simulink model "Huang_Isoherranen_Mechanistic_Kidney_Model"  (R2017b)
settings: Solver=VariableStepAuto  StartTime=0.0  StopTime=Tfinish  RelTol=1e-3  EnableMultiTasking=on
values from neighbouring files (symbols this model uses):
  alpha_1 = 1    [Huang_Isoherranen_Mechanistic_Kidney_Model_Example_Code.m]
  alpha_10 = 1    [Huang_Isoherranen_Mechanistic_Kidney_Model_Example_Code.m]
  alpha_11 = 1    [Huang_Isoherranen_Mechanistic_Kidney_Model_Example_Code.m]
  alpha_2 = 1    [Huang_Isoherranen_Mechanistic_Kidney_Model_Example_Code.m]
  alpha_3 = 1    [Huang_Isoherranen_Mechanistic_Kidney_Model_Example_Code.m]
  alpha_4 = 1    [Huang_Isoherranen_Mechanistic_Kidney_Model_Example_Code.m]
  alpha_5 = 1    [Huang_Isoherranen_Mechanistic_Kidney_Model_Example_Code.m]
  alpha_6 = 1    [Huang_Isoherranen_Mechanistic_Kidney_Model_Example_Code.m]
  alpha_7 = 1    [Huang_Isoherranen_Mechanistic_Kidney_Model_Example_Code.m]
  alpha_8 = 1    [Huang_Isoherranen_Mechanistic_Kidney_Model_Example_Code.m]
  alpha_9 = 1    [Huang_Isoherranen_Mechanistic_Kidney_Model_Example_Code.m]
  beta = 1    [Huang_Isoherranen_Mechanistic_Kidney_Model_Example_Code.m]
  BP0 = 1    [Huang_Isoherranen_Mechanistic_Kidney_Model_Example_Code.m]
  CL_api_reabs = 0    [Huang_Isoherranen_Mechanistic_Kidney_Model_Example_Code.m]
  CL_BC = 0    [Huang_Isoherranen_Mechanistic_Kidney_Model_Example_Code.m]
  CL_bsl_reabs = 0    [Huang_Isoherranen_Mechanistic_Kidney_Model_Example_Code.m]
  CL_CT = 0    [Huang_Isoherranen_Mechanistic_Kidney_Model_Example_Code.m]
  CL_kidney_intrinsic = 0    [Huang_Isoherranen_Mechanistic_Kidney_Model_Example_Code.m]
  CL_PD_CD = S_CD * Papp    (= 0.01608)    [Huang_Isoherranen_Mechanistic_Kidney_Model_Example_Code.m]
  CL_PD_DS = S_DT * Papp    (= 0.3744)    [Huang_Isoherranen_Mechanistic_Kidney_Model_Example_Code.m]
  CL_PD_LH = S_HT * Papp    (= 0.1464)    [Huang_Isoherranen_Mechanistic_Kidney_Model_Example_Code.m]
  CL_PD_PX_apical = S_PT * Papp    (= 14.6568)    [Huang_Isoherranen_Mechanistic_Kidney_Model_Example_Code.m]
  CL_PD_PX_basolateral = S_PT/30 * Papp    (= 0.48856)    [Huang_Isoherranen_Mechanistic_Kidney_Model_Example_Code.m]
  CLh = 0    [Huang_Isoherranen_Mechanistic_Kidney_Model_Example_Code.m]
  fu0 = 1    [Huang_Isoherranen_Mechanistic_Kidney_Model_Example_Code.m]
  fu_k = fu0    (= 1)    [Huang_Isoherranen_Mechanistic_Kidney_Model_Example_Code.m]
  gamma = 1    [Huang_Isoherranen_Mechanistic_Kidney_Model_Example_Code.m]
  Infusion_length = 240    [Huang_Isoherranen_Mechanistic_Kidney_Model_Example_Code.m]
  IR = 1    [Huang_Isoherranen_Mechanistic_Kidney_Model_Example_Code.m]
  ivbolusDose1 = 0    [Huang_Isoherranen_Mechanistic_Kidney_Model_Example_Code.m]
  ivT1 = 0    [Huang_Isoherranen_Mechanistic_Kidney_Model_Example_Code.m]
  Q_connectingtubule = 11    [Huang_Isoherranen_Mechanistic_Kidney_Model_Example_Code.m]
  Q_corticalCD = 7    [Huang_Isoherranen_Mechanistic_Kidney_Model_Example_Code.m]
  Q_GFR = 7.2    [Huang_Isoherranen_Mechanistic_Kidney_Model_Example_Code.m]
  Q_initialCD = 9    [Huang_Isoherranen_Mechanistic_Kidney_Model_Example_Code.m]
  Q_kidney0 = 60    [Huang_Isoherranen_Mechanistic_Kidney_Model_Example_Code.m]
  Q_medullaryCD = 5    [Huang_Isoherranen_Mechanistic_Kidney_Model_Example_Code.m]
  Q_papillary = 3    [Huang_Isoherranen_Mechanistic_Kidney_Model_Example_Code.m]
  Q_urine = 1    [Huang_Isoherranen_Mechanistic_Kidney_Model_Example_Code.m]
  Qc0 = 330    [Huang_Isoherranen_Mechanistic_Kidney_Model_Example_Code.m]
  Tstart_infusion = 0    [Huang_Isoherranen_Mechanistic_Kidney_Model_Example_Code.m]
  V_CDB = 0.237    [Huang_Isoherranen_Mechanistic_Kidney_Model_Example_Code.m]
  V_CDC = 0.237    [Huang_Isoherranen_Mechanistic_Kidney_Model_Example_Code.m]
  V_CDT = 0.237    [Huang_Isoherranen_Mechanistic_Kidney_Model_Example_Code.m]
  V_DB = 0.0194    [Huang_Isoherranen_Mechanistic_Kidney_Model_Example_Code.m]
  V_DC = 0.0194    [Huang_Isoherranen_Mechanistic_Kidney_Model_Example_Code.m]
  V_DT = 0.0194    [Huang_Isoherranen_Mechanistic_Kidney_Model_Example_Code.m]
  V_HB = 0.0027    [Huang_Isoherranen_Mechanistic_Kidney_Model_Example_Code.m]
  V_HC = 0.0027    [Huang_Isoherranen_Mechanistic_Kidney_Model_Example_Code.m]
  V_HT = 0.0027    [Huang_Isoherranen_Mechanistic_Kidney_Model_Example_Code.m]
  V_PB = 0.0305    [Huang_Isoherranen_Mechanistic_Kidney_Model_Example_Code.m]
  V_PC = 0.0305    [Huang_Isoherranen_Mechanistic_Kidney_Model_Example_Code.m]
  V_PT = 0.0305    [Huang_Isoherranen_Mechanistic_Kidney_Model_Example_Code.m]
  V_ven0 = 42    [Huang_Isoherranen_Mechanistic_Kidney_Model_Example_Code.m]
libraries: simulink x3, dspmathops x1
(part 1 of 2)
settings Model: Creator=Weize Huang  LastModifiedBy=isolab
settings SolverCC: MaxConsecutiveZCs=2000
settings OptimizationCC: LifeSpan=inf
settings DebuggingCC: SFUnexpectedBacktrackingDiag=warning  SFNoUnconditionalDefaultTransitionDiag=warning  SFExecutionAtInitializationDiag=none
settings CodeAppCC: StateflowObjectComments=on
settings GRTTargetCC: TargetLangStandard=C89/C90 (ANSI)  GeneratePreprocessorConditionals=Disable all
settings ConfigComp: CovMetricSettings=dw  CovHtmlReporting=on  CovSaveCumulativeToWorkspaceVar=on  CovSaveSingleToWorkspaceVar=on  CovExternalEMLEnable=off

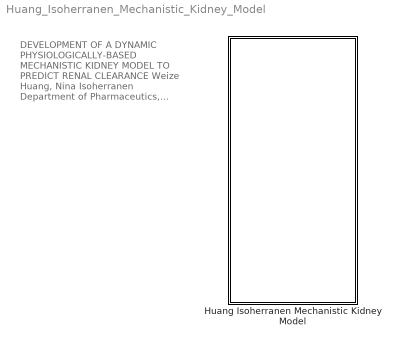
== system Huang_Isoherranen_Mechanistic_Kidney_Model ==
  note: DEVELOPMENT OF A DYNAMIC PHYSIOLOGICALLY-BASED MECHANISTIC KIDNEY MODEL TO PREDICT RENAL CLEARANCE
      | Weize Huang, Nina Isoherranen
      | Department of Pharmaceutics, School of Pharmacy, University of Washington, Seattle, WA, 98195
      | May 2nd 2018
  Huang Isoherranen Mechanistic Kidney Model : Subsystem

== system Huang_Isoherranen_Mechanistic_Kidney_Model/Huang Isoherranen Mechanistic Kidney Model ==
  note: DEVELOPMENT OF A DYNAMIC PHYSIOLOGICALLY-BASED MECHANISTIC KIDNEY MODEL TO PREDICT RENAL CLEARANCE
      | Weize Huang, Nina Isoherranen
      | Department of Pharmaceutics, School of Pharmacy, University of Washington, Seattle, WA, 98195
      | May 2nd 2018
  Kidney : Subsystem
  venous blood : Subsystem
  wires:
  Kidney/1(Out1) -> venous blood/2(In2)
  venous blood/1(Out1) -> Kidney/1(In1), venous blood/1(In1)

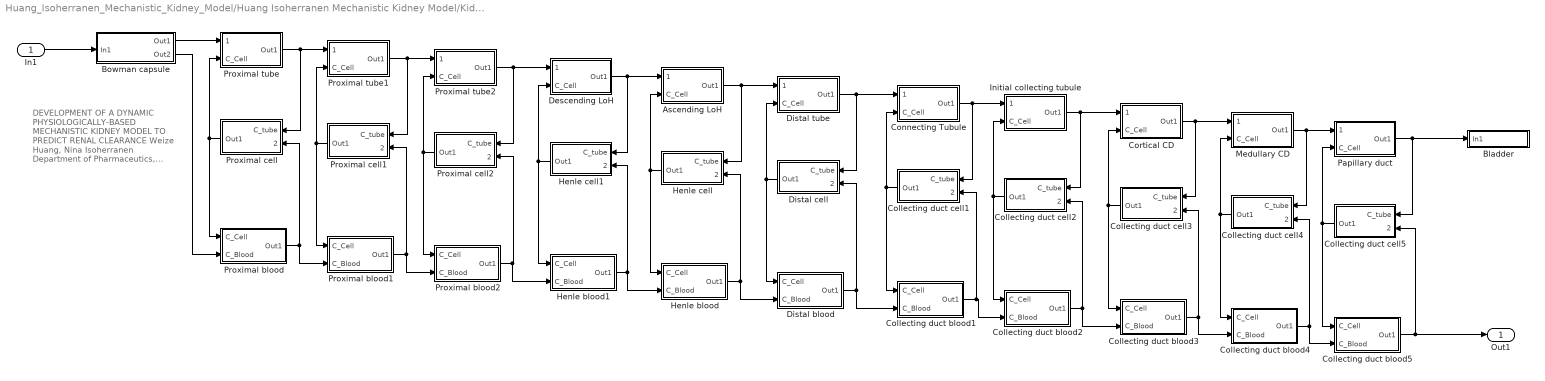
== system Huang_Isoherranen_Mechanistic_Kidney_Model/Huang Isoherranen Mechanistic Kidney Model/Kidney ==
  note: DEVELOPMENT OF A DYNAMIC PHYSIOLOGICALLY-BASED MECHANISTIC KIDNEY MODEL TO PREDICT RENAL CLEARANCE
      | Weize Huang, Nina Isoherranen
      | Department of Pharmaceutics, School of Pharmacy, University of Washington, Seattle, WA, 98195
      | May 2nd 2018
  In1 : Inport
  Ascending LoH : Subsystem
  Bladder : Subsystem
  Bowman capsule : Subsystem
  Collecting duct blood1 : Subsystem
  Collecting duct blood2 : Subsystem
  Collecting duct blood3 : Subsystem
  Collecting duct blood4 : Subsystem
  Collecting duct blood5 : Subsystem
  Collecting duct cell1 : Subsystem
  Collecting duct cell2 : Subsystem
  Collecting duct cell3 : Subsystem
  Collecting duct cell4 : Subsystem
  Collecting duct cell5 : Subsystem
  Connecting Tubule : Subsystem
  Cortical CD : Subsystem
  Descending LoH : Subsystem
  Distal blood : Subsystem
  Distal cell : Subsystem
  Distal tube : Subsystem
  Henle blood : Subsystem
  Henle blood1 : Subsystem
  Henle cell : Subsystem
  Henle cell1 : Subsystem
  Initial collecting tubule : Subsystem
  Medullary CD : Subsystem
  Papillary duct : Subsystem
  Proximal blood : Subsystem
  Proximal blood1 : Subsystem
  Proximal blood2 : Subsystem
  Proximal cell : Subsystem
  Proximal cell1 : Subsystem
  Proximal cell2 : Subsystem
  Proximal tube : Subsystem
  Proximal tube1 : Subsystem
  Proximal tube2 : Subsystem
  Out1 : Outport
  wires:
  In1/1 -> Bowman capsule/1(In1)
  Bowman capsule/1(Out1) -> Proximal tube/1(C_Tube)
  Proximal tube/1(Out1) -> Proximal tube1/1(C_Tube), Proximal cell/1(C_tube)
  Proximal cell/1(Out1) -> Proximal tube/2(C_Cell), Proximal blood/1(C_Cell)
  Proximal blood/1(Out1) -> Proximal blood1/2(C_Blood), Proximal cell/2(C_blood)
  Proximal tube1/1(Out1) -> Proximal cell1/1(C_tube), Proximal tube2/1(C_Tube)
  Proximal blood1/1(Out1) -> Proximal blood2/2(C_Blood), Proximal cell1/2(C_blood)
  Proximal tube2/1(Out1) -> Proximal cell2/1(C_tube), Descending LoH/1(C_Tube)
  Proximal blood2/1(Out1) -> Proximal cell2/2(C_blood), Henle blood1/2(C_Blood)
  Proximal cell1/1(Out1) -> Proximal blood1/1(C_Cell), Proximal tube1/2(C_Cell)
  Proximal cell2/1(Out1) -> Proximal blood2/1(C_Cell), Proximal tube2/2(C_Cell)
  Ascending LoH/1(Out1) -> Distal tube/1(C_Tube), Henle cell/1(C_tube)
  Henle cell/1(Out1) -> Henle blood/1(C_Cell), Ascending LoH/2(C_Cell)
  Henle blood/1(Out1) -> Distal blood/2(C_Blood), Henle cell/2(C_blood)
  Distal tube/1(Out1) -> Distal cell/1(C_tube), Connecting Tubule/1(C_Tube)
  Distal cell/1(Out1) -> Distal blood/1(C_Cell), Distal tube/2(C_Cell)
  Distal blood/1(Out1) -> Distal cell/2(C_blood), Collecting duct blood1/2(C_Blood)
  Collecting duct cell1/1(Out1) -> Collecting duct blood1/1(C_Cell), Connecting Tubule/2(C_Cell)
  Collecting duct cell4/1(Out1) -> Collecting duct blood4/1(C_Cell), Medullary CD/2(C_Cell)
  Collecting duct cell2/1(Out1) -> Collecting duct blood2/1(C_Cell), Initial collecting tubule/2(C_Cell)
  Collecting duct cell3/1(Out1) -> Collecting duct blood3/1(C_Cell), Cortical CD/2(C_Cell)
  Connecting Tubule/1(Out1) -> Collecting duct cell1/1(C_tube), Initial collecting tubule/1(C_Tube)
  Collecting duct blood1/1(Out1) -> Collecting duct cell1/2(C_blood), Collecting duct blood2/2(C_Blood)
  Initial collecting tubule/1(Out1) -> Collecting duct cell2/1(C_tube), Cortical CD/1(C_Tube)
  Collecting duct blood2/1(Out1) -> Collecting duct cell2/2(C_blood), Collecting duct blood3/2(C_Blood)
  Cortical CD/1(Out1) -> Collecting duct cell3/1(C_tube), Medullary CD/1(C_Tube)
  Collecting duct blood3/1(Out1) -> Collecting duct blood4/2(C_Blood), Collecting duct cell3/2(C_blood)
  Henle blood1/1(Out1) -> Henle cell1/2(C_blood), Henle blood/2(C_Blood)
  Papillary duct/1(Out1) -> Collecting duct cell5/1(C_tube), Bladder/1(In1)
  Collecting duct blood5/1(Out1) -> Collecting duct cell5/2(C_blood), Out1/1
  Collecting duct cell5/1(Out1) -> Collecting duct blood5/1(C_Cell), Papillary duct/2(C_Cell)
  Medullary CD/1(Out1) -> Collecting duct cell4/1(C_tube), Papillary duct/1(C_Tube)
  Collecting duct blood4/1(Out1) -> Collecting duct blood5/2(C_Blood), Collecting duct cell4/2(C_blood)
  Henle cell1/1(Out1) -> Henle blood1/1(C_Cell), Descending LoH/2(C_Cell)
  Descending LoH/1(Out1) -> Henle cell1/1(C_tube), Ascending LoH/1(C_Tube)
  Bowman capsule/2(Out2) -> Proximal blood/2(C_Blood)

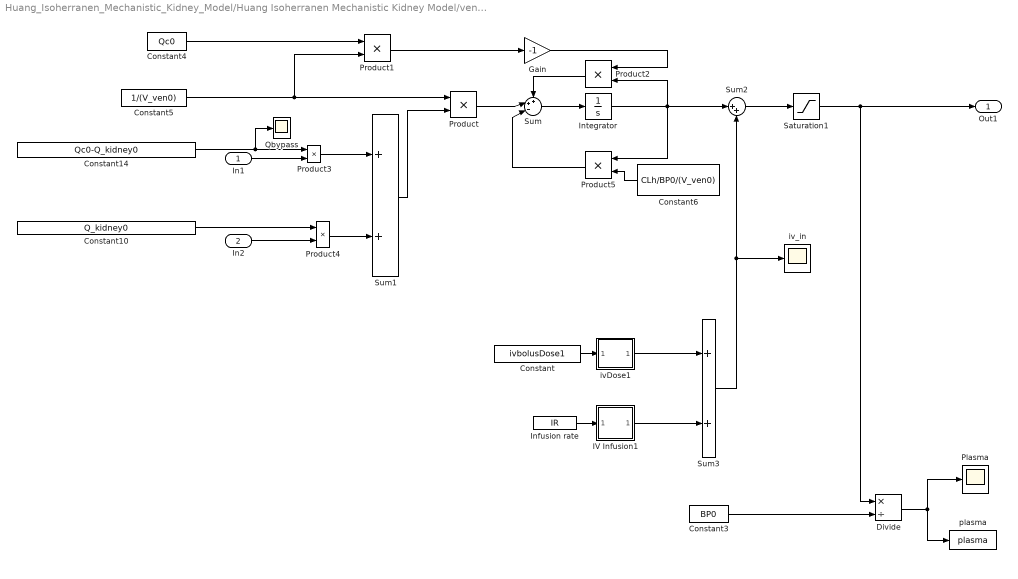
== system Huang_Isoherranen_Mechanistic_Kidney_Model/Huang Isoherranen Mechanistic Kidney Model/venous blood ==
  In1 : Inport
  In2 : Inport  Port=2
  Constant : Constant  Value=ivbolusDose1
  Constant10 : Constant  Value=Q_kidney0
  Constant14 : Constant  Value=Qc0-Q_kidney0
  Constant3 : Constant  Value=BP0
  Constant4 : Constant  Value=Qc0
  Constant5 : Constant  Value=1/(V_ven0)
  Constant6 : Constant  Value=CLh/BP0/(V_ven0)
  Divide : Product  Inputs=*/
  Gain : Gain  Gain=-1
  IV Infusion1 : Subsystem
  Infusion rate : Constant  Value=IR
  Integrator : Integrator
  Plasma : Scope
  Product{,1..5} (6 alike) : Product  RndMeth=Zero
  Qbypass : Scope
  Saturation1 : Saturate  UpperLimit=1000000000  LowerLimit=0
  Sum : Sum  Inputs=++-|
  Sum1 : Sum
  Sum2 : Sum  Inputs=|++
  Sum3 : Sum
  ivDose1 : Subsystem
  iv_in : Scope
  plasma : ToWorkspace  VariableName=plasma  SampleTime=-1
  Out1 : Outport
  wires:
  Product1/1 -> Gain/1
  Product2/1 -> Sum/1
  Product/1 -> Sum/2
  Sum/1 -> Integrator/1
  Gain/1 -> Product2/1
  Sum1/1 -> Product/2
  Sum2/1 -> Saturation1/1
  Product3/1 -> Sum1/1
  Product4/1 -> Sum1/2
  Divide/1 -> plasma/1, Plasma/1
  Constant3/1 -> Divide/2
  Constant10/1 -> Product4/1
  Constant14/1 -> Qbypass/1, Product3/1
  Constant5/1 -> Product/1, Product1/2
  Integrator/1 -> Product5/1, Sum2/1, Product2/2
  Constant4/1 -> Product1/1
  Constant/1 -> ivDose1/1(In1)
  Sum3/1 -> Sum2/2, iv_in/1
  ivDose1/1(Out1) -> Sum3/1
  Saturation1/1 -> Out1/1, Divide/1
  In1/1 -> Product3/2
  In2/1 -> Product4/2
  Constant6/1 -> Product5/2
  Product5/1 -> Sum/3
  Infusion rate/1 -> IV Infusion1/1(In1)
  IV Infusion1/1(Out1) -> Sum3/2

== system Huang_Isoherranen_Mechanistic_Kidney_Model/Huang Isoherranen Mechanistic Kidney Model/Kidney/Ascending LoH ==
  C_Tube : Inport
  C_Cell : Inport  Port=2
  C_HT : ToWorkspace  VariableName=C_HT_2  SampleTime=-1
  Constant1 : Constant  Value=V_HT
  Constant2 : Constant  Value=CL_PD_LH
  Constant3 : Constant  Value=beta
  Constant4 : Constant  Value=Q_GFR/120*24
  Constant5 : Constant  Value=Q_GFR/120*24
  Constant6 : Constant  Value=alpha_5
  Constant7 : Constant  Value=fu_k
  Divide1 : Product  Inputs=/*
  Integrator : Integrator
  Product{,1..3,5} (5 alike) : Product  RndMeth=Zero
  Product6 : Product  Inputs=3  RndMeth=Zero
  Saturation : Saturate  UpperLimit=1000000000  LowerLimit=0
  Subtract : Sum
  Subtract1 : Sum
  Sum : Sum  Inputs=+-|
  scope : Scope
  Out1 : Outport
  wires:
  Integrator/1 -> Product2/2, Product6/3, Saturation/1, scope/1, C_HT/1
  Sum/1 -> Divide1/2
  Saturation/1 -> Out1/1
  C_Tube/1 -> Product/2
  Constant7/1 -> Product1/1
  C_Cell/1 -> Product1/2
  Product1/1 -> Product3/1
  Constant5/1 -> Product/1
  Product3/1 -> Subtract/1
  Product/1 -> Subtract/2
  Constant1/1 -> Divide1/1
  Subtract/1 -> Sum/1
  Divide1/1 -> Integrator/1
  Constant4/1 -> Product2/1
  Constant3/1 -> Product5/1
  Constant2/1 -> Product6/2, Product5/2
  Product5/1 -> Product3/2
  Constant6/1 -> Product6/1
  Product6/1 -> Subtract1/1
  Product2/1 -> Subtract1/2
  Subtract1/1 -> Sum/2

== system Huang_Isoherranen_Mechanistic_Kidney_Model/Huang Isoherranen Mechanistic Kidney Model/Kidney/Bladder ==
  In1 : Inport
  Ae : ToWorkspace  VariableName=Ae  SampleTime=-1
  C_bladder_urine : ToWorkspace  VariableName=C_bladder_urine  SampleTime=-1
  Constant4 : Constant  Value=Q_GFR/120*Q_urine
  Cum_Ae : ToWorkspace  VariableName=Cum_Ae  SampleTime=-1
  Cumulative Sum : dspmathops/Cumulative Sum  dim=Columns  InputProcessing=Columns as channels (frame based)  reset_popup=None  outputDataTypeStr=Inherit: Same as accumulator  outputLastDataTypeStr=Inherit: Same as accumulator  outputMin=[]  outputMax=[]  roundingMode=Floor  overflowMode=off
      settings: SourceProductName=DSP System Toolbox
  Gain : Gain
  Integrator : Integrator
  Product2 : Product  RndMeth=Zero
  scope : Scope
  wires:
  In1/1 -> Gain/1
  Gain/1 -> Product2/1, scope/1, C_bladder_urine/1
  Constant4/1 -> Product2/2
  Product2/1 -> Integrator/1
  Integrator/1 -> Cumulative Sum/1, Ae/1
  Cumulative Sum/1 -> Cum_Ae/1

== system Huang_Isoherranen_Mechanistic_Kidney_Model/Huang Isoherranen Mechanistic Kidney Model/Kidney/Bowman capsule ==
  In1 : Inport
  Bowman : ToWorkspace  VariableName=Bowman  SampleTime=-1
  Constant : Constant  Value=fu0/BP0
  Constant1 : Constant  Value=1-fu0/BP0*Q_GFR/Q_kidney0
  Product1 : Product  RndMeth=Zero
  Product2 : Product  RndMeth=Zero
  Saturation : Saturate  UpperLimit=1000000000  LowerLimit=0
  blood_after_filtration : ToWorkspace  VariableName=C_blood_after_filtration1  SampleTime=-1
  scope : Scope
  scope1 : Scope
  Out1 : Outport
  Out2 : Outport  Port=2
  wires:
  Product1/1 -> scope/1, Bowman/1, Saturation/1
  Saturation/1 -> Out1/1
  In1/1 -> Product2/2, Product1/1
  Constant/1 -> Product1/2
  Product2/1 -> Out2/1, scope1/1, blood_after_filtration/1
  Constant1/1 -> Product2/1

== system Huang_Isoherranen_Mechanistic_Kidney_Model/Huang Isoherranen Mechanistic Kidney Model/Kidney/Collecting duct blood1 ==
  C_Cell : Inport
  C_Blood : Inport  Port=2
  C_CDB_1 : ToWorkspace  VariableName=C_CDB  SampleTime=-1
  Constant : Constant  Value=fu0/BP0
  Constant1 : Constant  Value=V_CDB
  Constant2 : Constant  Value=CL_PD_CD
  Constant3 : Constant  Value=beta
  Constant5 : Constant  Value=Q_kidney0
  Constant6 : Constant  Value=gamma
  Constant7 : Constant  Value=fu_k
  Divide1 : Product  Inputs=/*
  Integrator : Integrator
  Product{,1..3,5} (5 alike) : Product  RndMeth=Zero
  Product6 : Product  Inputs=4  RndMeth=Zero
  Saturation : Saturate  UpperLimit=1000000000  LowerLimit=0
  Subtract : Sum
  Subtract1 : Sum
  Sum : Sum  Inputs=+-|
  scope : Scope
  Out1 : Outport
  wires:
  Integrator/1 -> Product2/2, Product6/4, Saturation/1, scope/1, C_CDB_1/1
  Sum/1 -> Divide1/2
  Saturation/1 -> Out1/1
  Constant7/1 -> Product1/1
  Product1/1 -> Product3/1
  Constant5/1 -> Product2/1, Product/1
  Product3/1 -> Subtract/1
  Product/1 -> Subtract/2
  Constant1/1 -> Divide1/1
  Subtract/1 -> Sum/1
  Divide1/1 -> Integrator/1
  Constant3/1 -> Product5/1
  Constant2/1 -> Product6/3, Product5/2
  Product5/1 -> Product3/2
  Subtract1/1 -> Sum/2
  C_Cell/1 -> Product1/2
  C_Blood/1 -> Product/2
  Constant/1 -> Product6/1
  Product2/1 -> Subtract1/1
  Constant6/1 -> Product6/2
  Product6/1 -> Subtract1/2

== system Huang_Isoherranen_Mechanistic_Kidney_Model/Huang Isoherranen Mechanistic Kidney Model/Kidney/Collecting duct blood2 ==
  C_Cell : Inport
  C_Blood : Inport  Port=2
  C_CDB_2 : ToWorkspace  VariableName=C_CDB_2  SampleTime=-1
  Constant : Constant  Value=fu0/BP0
  Constant1 : Constant  Value=V_CDB
  Constant2 : Constant  Value=CL_PD_CD
  Constant3 : Constant  Value=beta
  Constant5 : Constant  Value=Q_kidney0
  Constant6 : Constant  Value=gamma
  Constant7 : Constant  Value=fu_k
  Divide1 : Product  Inputs=/*
  Integrator : Integrator
  Product{,1..3,5} (5 alike) : Product  RndMeth=Zero
  Product6 : Product  Inputs=4  RndMeth=Zero
  Saturation : Saturate  UpperLimit=1000000000  LowerLimit=0
  Subtract : Sum
  Subtract1 : Sum
  Sum : Sum  Inputs=+-|
  scope : Scope
  Out1 : Outport
  wires:
  Integrator/1 -> Product2/2, Product6/4, Saturation/1, scope/1, C_CDB_2/1
  Sum/1 -> Divide1/2
  Saturation/1 -> Out1/1
  Constant7/1 -> Product1/1
  Product1/1 -> Product3/1
  Constant5/1 -> Product2/1, Product/1
  Product3/1 -> Subtract/1
  Product/1 -> Subtract/2
  Constant1/1 -> Divide1/1
  Subtract/1 -> Sum/1
  Divide1/1 -> Integrator/1
  Constant3/1 -> Product5/1
  Constant2/1 -> Product6/3, Product5/2
  Product5/1 -> Product3/2
  Subtract1/1 -> Sum/2
  C_Cell/1 -> Product1/2
  C_Blood/1 -> Product/2
  Constant/1 -> Product6/1
  Product2/1 -> Subtract1/1
  Constant6/1 -> Product6/2
  Product6/1 -> Subtract1/2

== system Huang_Isoherranen_Mechanistic_Kidney_Model/Huang Isoherranen Mechanistic Kidney Model/Kidney/Collecting duct blood3 ==
  C_Cell : Inport
  C_Blood : Inport  Port=2
  C_CDB_3 : ToWorkspace  VariableName=C_CDB_3  SampleTime=-1
  Constant : Constant  Value=fu0/BP0
  Constant1 : Constant  Value=V_CDB
  Constant2 : Constant  Value=CL_PD_CD
  Constant3 : Constant  Value=beta
  Constant5 : Constant  Value=Q_kidney0
  Constant6 : Constant  Value=gamma
  Constant7 : Constant  Value=fu_k
  Divide1 : Product  Inputs=/*
  Integrator : Integrator
  Product{,1..3,5} (5 alike) : Product  RndMeth=Zero
  Product6 : Product  Inputs=4  RndMeth=Zero
  Saturation : Saturate  UpperLimit=1000000000  LowerLimit=0
  Subtract : Sum
  Subtract1 : Sum
  Sum : Sum  Inputs=+-|
  scope : Scope
  Out1 : Outport
  wires:
  Integrator/1 -> Product2/2, Product6/4, Saturation/1, scope/1, C_CDB_3/1
  Sum/1 -> Divide1/2
  Saturation/1 -> Out1/1
  Constant7/1 -> Product1/1
  Product1/1 -> Product3/1
  Constant5/1 -> Product2/1, Product/1
  Product3/1 -> Subtract/1
  Product/1 -> Subtract/2
  Constant1/1 -> Divide1/1
  Subtract/1 -> Sum/1
  Divide1/1 -> Integrator/1
  Constant3/1 -> Product5/1
  Constant2/1 -> Product6/3, Product5/2
  Product5/1 -> Product3/2
  Subtract1/1 -> Sum/2
  C_Cell/1 -> Product1/2
  C_Blood/1 -> Product/2
  Constant/1 -> Product6/1
  Product2/1 -> Subtract1/1
  Constant6/1 -> Product6/2
  Product6/1 -> Subtract1/2

== system Huang_Isoherranen_Mechanistic_Kidney_Model/Huang Isoherranen Mechanistic Kidney Model/Kidney/Collecting duct blood4 ==
  C_Cell : Inport
  C_Blood : Inport  Port=2
  C_CDB_4 : ToWorkspace  VariableName=C_CDB_4  SampleTime=-1
  Constant : Constant  Value=fu0/BP0
  Constant1 : Constant  Value=V_CDB
  Constant2 : Constant  Value=CL_PD_CD
  Constant3 : Constant  Value=beta
  Constant5 : Constant  Value=Q_kidney0
  Constant6 : Constant  Value=gamma
  Constant7 : Constant  Value=fu_k
  Divide1 : Product  Inputs=/*
  Integrator : Integrator
  Product{,1..3,5} (5 alike) : Product  RndMeth=Zero
  Product6 : Product  Inputs=4  RndMeth=Zero
  Saturation : Saturate  UpperLimit=1000000000  LowerLimit=0
  Subtract : Sum
  Subtract1 : Sum
  Sum : Sum  Inputs=+-|
  scope : Scope
  Out1 : Outport
  wires:
  Integrator/1 -> Product2/2, Product6/4, Saturation/1, scope/1, C_CDB_4/1
  Sum/1 -> Divide1/2
  Saturation/1 -> Out1/1
  Constant7/1 -> Product1/1
  Product1/1 -> Product3/1
  Constant5/1 -> Product2/1, Product/1
  Product3/1 -> Subtract/1
  Product/1 -> Subtract/2
  Constant1/1 -> Divide1/1
  Subtract/1 -> Sum/1
  Divide1/1 -> Integrator/1
  Constant3/1 -> Product5/1
  Constant2/1 -> Product6/3, Product5/2
  Product5/1 -> Product3/2
  Subtract1/1 -> Sum/2
  C_Cell/1 -> Product1/2
  C_Blood/1 -> Product/2
  Constant/1 -> Product6/1
  Product2/1 -> Subtract1/1
  Constant6/1 -> Product6/2
  Product6/1 -> Subtract1/2

== system Huang_Isoherranen_Mechanistic_Kidney_Model/Huang Isoherranen Mechanistic Kidney Model/Kidney/Collecting duct blood5 ==
  C_Cell : Inport
  C_Blood : Inport  Port=2
  C_CDB_4 : ToWorkspace  VariableName=C_CDB_5  SampleTime=-1
  Constant : Constant  Value=fu0/BP0
  Constant1 : Constant  Value=V_CDB
  Constant2 : Constant  Value=CL_PD_CD
  Constant3 : Constant  Value=beta
  Constant5 : Constant  Value=Q_kidney0
  Constant6 : Constant  Value=gamma
  Constant7 : Constant  Value=fu_k
  Divide1 : Product  Inputs=/*
  Integrator : Integrator
  Product{,1..3,5} (5 alike) : Product  RndMeth=Zero
  Product6 : Product  Inputs=4  RndMeth=Zero
  Saturation : Saturate  UpperLimit=1000000000  LowerLimit=0
  Subtract : Sum
  Subtract1 : Sum
  Sum : Sum  Inputs=+-|
  scope : Scope
  Out1 : Outport
  wires:
  Integrator/1 -> Product2/2, Product6/4, Saturation/1, scope/1, C_CDB_4/1
  Sum/1 -> Divide1/2
  Saturation/1 -> Out1/1
  Constant7/1 -> Product1/1
  Product1/1 -> Product3/1
  Constant5/1 -> Product2/1, Product/1
  Product3/1 -> Subtract/1
  Product/1 -> Subtract/2
  Constant1/1 -> Divide1/1
  Subtract/1 -> Sum/1
  Divide1/1 -> Integrator/1
  Constant3/1 -> Product5/1
  Constant2/1 -> Product6/3, Product5/2
  Product5/1 -> Product3/2
  Subtract1/1 -> Sum/2
  C_Cell/1 -> Product1/2
  C_Blood/1 -> Product/2
  Constant/1 -> Product6/1
  Product2/1 -> Subtract1/1
  Constant6/1 -> Product6/2
  Product6/1 -> Subtract1/2

== system Huang_Isoherranen_Mechanistic_Kidney_Model/Huang Isoherranen Mechanistic Kidney Model/Kidney/Collecting duct cell1 ==
  C_tube : Inport
  C_blood : Inport  Port=2
  C_CDC_1 : ToWorkspace  VariableName=C_CDC  SampleTime=-1
  Constant : Constant  Value=CL_PD_CD
  Constant1 : Constant  Value=V_CDC
  Constant2 : Constant  Value=CL_PD_CD
  Constant3 : Constant  Value=fu0/BP0
  Constant4 : Constant  Value=gamma
  Constant6 : Constant  Value=alpha_7
  Constant7 : Constant  Value=fu_k
  Constant8 : Constant  Value=beta
  Divide2 : Product  Inputs=/*
  Integrator : Integrator
  Product1 : Product  Inputs=3  RndMeth=Zero
  Product2 : Product  RndMeth=Zero
  Product3 : Product  Inputs=3  RndMeth=Zero
  Product4 : Product  RndMeth=Zero
  Product7 : Product  Inputs=3  RndMeth=Zero
  Subtract : Sum
  Subtract1 : Sum
  Sum : Sum  Inputs=+-|
  scope : Scope
  Out1 : Outport
  wires:
  Integrator/1 -> Product2/2, Out1/1, scope/1, C_CDC_1/1
  C_tube/1 -> Product1/2
  Constant/1 -> Subtract1/2, Product1/1
  Constant2/1 -> Subtract1/1, Product3/1
  Constant4/1 -> Product3/2
  Subtract/1 -> Sum/1
  Product3/1 -> Subtract/2
  C_blood/1 -> Product4/1
  Constant3/1 -> Product4/2
  Product4/1 -> Product3/3
  Constant6/1 -> Product1/3
  Product1/1 -> Subtract/1
  Sum/1 -> Divide2/2
  Constant1/1 -> Divide2/1
  Divide2/1 -> Integrator/1
  Product2/1 -> Product7/3
  Constant7/1 -> Product2/1
  Constant8/1 -> Product7/2
  Subtract1/1 -> Product7/1
  Product7/1 -> Sum/2

== system Huang_Isoherranen_Mechanistic_Kidney_Model/Huang Isoherranen Mechanistic Kidney Model/Kidney/Collecting duct cell2 ==
  C_tube : Inport
  C_blood : Inport  Port=2
  C_CDC_2 : ToWorkspace  VariableName=C_CDC_2  SampleTime=-1
  Constant : Constant  Value=CL_PD_CD
  Constant1 : Constant  Value=V_CDC
  Constant2 : Constant  Value=CL_PD_CD
  Constant3 : Constant  Value=fu0/BP0
  Constant4 : Constant  Value=gamma
  Constant6 : Constant  Value=alpha_8
  Constant7 : Constant  Value=fu_k
  Constant8 : Constant  Value=beta
  Divide2 : Product  Inputs=/*
  Integrator : Integrator
  Product1 : Product  Inputs=3  RndMeth=Zero
  Product2 : Product  RndMeth=Zero
  Product3 : Product  Inputs=3  RndMeth=Zero
  Product4 : Product  RndMeth=Zero
  Product7 : Product  Inputs=3  RndMeth=Zero
  Subtract : Sum
  Subtract1 : Sum
  Sum : Sum  Inputs=+-|
  scope : Scope
  Out1 : Outport
  wires:
  Integrator/1 -> Product2/2, Out1/1, scope/1, C_CDC_2/1
  C_tube/1 -> Product1/2
  Constant/1 -> Subtract1/2, Product1/1
  Constant2/1 -> Subtract1/1, Product3/1
  Constant4/1 -> Product3/2
  Subtract/1 -> Sum/1
  Product3/1 -> Subtract/2
  C_blood/1 -> Product4/1
  Constant3/1 -> Product4/2
  Product4/1 -> Product3/3
  Constant6/1 -> Product1/3
  Product1/1 -> Subtract/1
  Sum/1 -> Divide2/2
  Constant1/1 -> Divide2/1
  Divide2/1 -> Integrator/1
  Product2/1 -> Product7/3
  Constant7/1 -> Product2/1
  Constant8/1 -> Product7/2
  Subtract1/1 -> Product7/1
  Product7/1 -> Sum/2

== system Huang_Isoherranen_Mechanistic_Kidney_Model/Huang Isoherranen Mechanistic Kidney Model/Kidney/Collecting duct cell3 ==
  C_tube : Inport
  C_blood : Inport  Port=2
  C_CDC_3 : ToWorkspace  VariableName=C_CDC_3  SampleTime=-1
  Constant : Constant  Value=CL_PD_CD
  Constant1 : Constant  Value=V_CDC
  Constant2 : Constant  Value=CL_PD_CD
  Constant3 : Constant  Value=fu0/BP0
  Constant4 : Constant  Value=gamma
  Constant6 : Constant  Value=alpha_9
  Constant7 : Constant  Value=fu_k
  Constant8 : Constant  Value=beta
  Divide2 : Product  Inputs=/*
  Integrator : Integrator
  Product1 : Product  Inputs=3  RndMeth=Zero
  Product2 : Product  RndMeth=Zero
  Product3 : Product  Inputs=3  RndMeth=Zero
  Product4 : Product  RndMeth=Zero
  Product7 : Product  Inputs=3  RndMeth=Zero
  Subtract : Sum
  Subtract1 : Sum
  Sum : Sum  Inputs=+-|
  scope : Scope
  Out1 : Outport
  wires:
  Integrator/1 -> Product2/2, Out1/1, scope/1, C_CDC_3/1
  C_tube/1 -> Product1/2
  Constant/1 -> Subtract1/2, Product1/1
  Constant2/1 -> Subtract1/1, Product3/1
  Constant4/1 -> Product3/2
  Subtract/1 -> Sum/1
  Product3/1 -> Subtract/2
  C_blood/1 -> Product4/1
  Constant3/1 -> Product4/2
  Product4/1 -> Product3/3
  Constant6/1 -> Product1/3
  Product1/1 -> Subtract/1
  Sum/1 -> Divide2/2
  Constant1/1 -> Divide2/1
  Divide2/1 -> Integrator/1
  Product2/1 -> Product7/3
  Constant7/1 -> Product2/1
  Constant8/1 -> Product7/2
  Subtract1/1 -> Product7/1
  Product7/1 -> Sum/2

== system Huang_Isoherranen_Mechanistic_Kidney_Model/Huang Isoherranen Mechanistic Kidney Model/Kidney/Collecting duct cell4 ==
  C_tube : Inport
  C_blood : Inport  Port=2
  C_CDC_4 : ToWorkspace  VariableName=C_CDC_4  SampleTime=-1
  Constant : Constant  Value=CL_PD_CD
  Constant1 : Constant  Value=V_CDC
  Constant2 : Constant  Value=CL_PD_CD
  Constant3 : Constant  Value=fu0/BP0
  Constant4 : Constant  Value=gamma
  Constant6 : Constant  Value=alpha_10
  Constant7 : Constant  Value=fu_k
  Constant8 : Constant  Value=beta
  Divide2 : Product  Inputs=/*
  Integrator : Integrator
  Product1 : Product  Inputs=3  RndMeth=Zero
  Product2 : Product  RndMeth=Zero
  Product3 : Product  Inputs=3  RndMeth=Zero
  Product4 : Product  RndMeth=Zero
  Product7 : Product  Inputs=3  RndMeth=Zero
  Subtract : Sum
  Subtract1 : Sum
  Sum : Sum  Inputs=+-|
  scope : Scope
  Out1 : Outport
  wires:
  Integrator/1 -> Product2/2, Out1/1, scope/1, C_CDC_4/1
  C_tube/1 -> Product1/2
  Constant/1 -> Subtract1/2, Product1/1
  Constant2/1 -> Subtract1/1, Product3/1
  Constant4/1 -> Product3/2
  Subtract/1 -> Sum/1
  Product3/1 -> Subtract/2
  C_blood/1 -> Product4/1
  Constant3/1 -> Product4/2
  Product4/1 -> Product3/3
  Constant6/1 -> Product1/3
  Product1/1 -> Subtract/1
  Sum/1 -> Divide2/2
  Constant1/1 -> Divide2/1
  Divide2/1 -> Integrator/1
  Product2/1 -> Product7/3
  Constant7/1 -> Product2/1
  Constant8/1 -> Product7/2
  Subtract1/1 -> Product7/1
  Product7/1 -> Sum/2

== system Huang_Isoherranen_Mechanistic_Kidney_Model/Huang Isoherranen Mechanistic Kidney Model/Kidney/Collecting duct cell5 ==
  C_tube : Inport
  C_blood : Inport  Port=2
  C_CDC_4 : ToWorkspace  VariableName=C_CDC_5  SampleTime=-1
  Constant : Constant  Value=CL_PD_CD
  Constant1 : Constant  Value=V_CDC
  Constant2 : Constant  Value=CL_PD_CD
  Constant3 : Constant  Value=fu0/BP0
  Constant4 : Constant  Value=gamma
  Constant6 : Constant  Value=alpha_11
  Constant7 : Constant  Value=fu_k
  Constant8 : Constant  Value=beta
  Divide2 : Product  Inputs=/*
  Integrator : Integrator
  Product1 : Product  Inputs=3  RndMeth=Zero
  Product2 : Product  RndMeth=Zero
  Product3 : Product  Inputs=3  RndMeth=Zero
  Product4 : Product  RndMeth=Zero
  Product7 : Product  Inputs=3  RndMeth=Zero
  Subtract : Sum
  Subtract1 : Sum
  Sum : Sum  Inputs=+-|
  scope : Scope
  Out1 : Outport
  wires:
  Integrator/1 -> Product2/2, Out1/1, scope/1, C_CDC_4/1
  C_tube/1 -> Product1/2
  Constant/1 -> Subtract1/2, Product1/1
  Constant2/1 -> Subtract1/1, Product3/1
  Constant4/1 -> Product3/2
  Subtract/1 -> Sum/1
  Product3/1 -> Subtract/2
  C_blood/1 -> Product4/1
  Constant3/1 -> Product4/2
  Product4/1 -> Product3/3
  Constant6/1 -> Product1/3
  Product1/1 -> Subtract/1
  Sum/1 -> Divide2/2
  Constant1/1 -> Divide2/1
  Divide2/1 -> Integrator/1
  Product2/1 -> Product7/3
  Constant7/1 -> Product2/1
  Constant8/1 -> Product7/2
  Subtract1/1 -> Product7/1
  Product7/1 -> Sum/2

== system Huang_Isoherranen_Mechanistic_Kidney_Model/Huang Isoherranen Mechanistic Kidney Model/Kidney/Connecting Tubule ==
  C_Tube : Inport
  C_Cell : Inport  Port=2
  C_CDT_1 : ToWorkspace  VariableName=C_CDT  SampleTime=-1
  Constant1 : Constant  Value=V_CDT
  Constant2 : Constant  Value=CL_PD_CD
  Constant3 : Constant  Value=beta
  Constant4 : Constant  Value=Q_GFR/120*Q_initialCD
  Constant5 : Constant  Value=Q_GFR/120*Q_connectingtubule
  Constant6 : Constant  Value=alpha_7
  Constant7 : Constant  Value=fu_k
  Divide1 : Product  Inputs=/*
  Integrator : Integrator
  Product{,1..3,5} (5 alike) : Product  RndMeth=Zero
  Product6 : Product  Inputs=3  RndMeth=Zero
  Saturation : Saturate  UpperLimit=1000000000  LowerLimit=0
  Subtract : Sum
  Subtract1 : Sum
  Sum : Sum  Inputs=+-|
  scope : Scope
  Out1 : Outport
  wires:
  Integrator/1 -> Product2/2, Product6/3, Saturation/1, scope/1, C_CDT_1/1
  Sum/1 -> Divide1/2
  Saturation/1 -> Out1/1
  C_Tube/1 -> Product/2
  Constant7/1 -> Product1/1
  C_Cell/1 -> Product1/2
  Product1/1 -> Product3/1
  Constant5/1 -> Product/1
  Product3/1 -> Subtract/1
  Product/1 -> Subtract/2
  Constant1/1 -> Divide1/1
  Subtract/1 -> Sum/1
  Divide1/1 -> Integrator/1
  Constant4/1 -> Product2/1
  Constant3/1 -> Product5/1
  Constant2/1 -> Product6/2, Product5/2
  Product5/1 -> Product3/2
  Constant6/1 -> Product6/1
  Product6/1 -> Subtract1/1
  Product2/1 -> Subtract1/2
  Subtract1/1 -> Sum/2

== system Huang_Isoherranen_Mechanistic_Kidney_Model/Huang Isoherranen Mechanistic Kidney Model/Kidney/Cortical CD ==
  C_Tube : Inport
  C_Cell : Inport  Port=2
  C_CDT_3 : ToWorkspace  VariableName=C_CDT_3  SampleTime=-1
  Constant1 : Constant  Value=V_CDT
  Constant2 : Constant  Value=CL_PD_CD
  Constant3 : Constant  Value=beta
  Constant4 : Constant  Value=Q_GFR/120*Q_medullaryCD
  Constant5 : Constant  Value=Q_GFR/120*Q_corticalCD
  Constant6 : Constant  Value=alpha_9
  Constant7 : Constant  Value=fu_k
  Divide1 : Product  Inputs=/*
  Integrator : Integrator
  Product{,1..3,5} (5 alike) : Product  RndMeth=Zero
  Product6 : Product  Inputs=3  RndMeth=Zero
  Saturation : Saturate  UpperLimit=1000000000  LowerLimit=0
  Subtract : Sum
  Subtract1 : Sum
  Sum : Sum  Inputs=+-|
  scope : Scope
  Out1 : Outport
  wires:
  Integrator/1 -> Product2/2, Product6/3, Saturation/1, scope/1, C_CDT_3/1
  Sum/1 -> Divide1/2
  Saturation/1 -> Out1/1
  C_Tube/1 -> Product/2
  Constant7/1 -> Product1/1
  C_Cell/1 -> Product1/2
  Product1/1 -> Product3/1
  Constant5/1 -> Product/1
  Product3/1 -> Subtract/1
  Product/1 -> Subtract/2
  Constant1/1 -> Divide1/1
  Subtract/1 -> Sum/1
  Divide1/1 -> Integrator/1
  Constant4/1 -> Product2/1
  Constant3/1 -> Product5/1
  Constant2/1 -> Product6/2, Product5/2
  Product5/1 -> Product3/2
  Constant6/1 -> Product6/1
  Product6/1 -> Subtract1/1
  Product2/1 -> Subtract1/2
  Subtract1/1 -> Sum/2

== system Huang_Isoherranen_Mechanistic_Kidney_Model/Huang Isoherranen Mechanistic Kidney Model/Kidney/Descending LoH ==
  C_Tube : Inport
  C_Cell : Inport  Port=2
  C_HT : ToWorkspace  VariableName=C_HT  SampleTime=-1
  Constant1 : Constant  Value=V_HT
  Constant2 : Constant  Value=CL_PD_LH
  Constant3 : Constant  Value=beta
  Constant4 : Constant  Value=Q_GFR/120*24
  Constant5 : Constant  Value=Q_GFR/120*43
  Constant6 : Constant  Value=alpha_4
  Constant7 : Constant  Value=fu_k
  Divide1 : Product  Inputs=/*
  Integrator : Integrator
  Product{,1..3,5} (5 alike) : Product  RndMeth=Zero
  Product6 : Product  Inputs=3  RndMeth=Zero
  Saturation : Saturate  UpperLimit=1000000000  LowerLimit=0
  Subtract : Sum
  Subtract1 : Sum
  Sum : Sum  Inputs=+-|
  scope : Scope
  Out1 : Outport
  wires:
  Integrator/1 -> Product2/2, Product6/3, Saturation/1, scope/1, C_HT/1
  Sum/1 -> Divide1/2
  Saturation/1 -> Out1/1
  C_Tube/1 -> Product/2
  Constant7/1 -> Product1/1
  C_Cell/1 -> Product1/2
  Product1/1 -> Product3/1
  Constant5/1 -> Product/1
  Product3/1 -> Subtract/1
  Product/1 -> Subtract/2
  Constant1/1 -> Divide1/1
  Subtract/1 -> Sum/1
  Divide1/1 -> Integrator/1
  Constant4/1 -> Product2/1
  Constant3/1 -> Product5/1
  Constant2/1 -> Product6/2, Product5/2
  Product5/1 -> Product3/2
  Constant6/1 -> Product6/1
  Product6/1 -> Subtract1/1
  Product2/1 -> Subtract1/2
  Subtract1/1 -> Sum/2

== system Huang_Isoherranen_Mechanistic_Kidney_Model/Huang Isoherranen Mechanistic Kidney Model/Kidney/Distal blood ==
  C_Cell : Inport
  C_Blood : Inport  Port=2
  C_DB : ToWorkspace  VariableName=C_DB  SampleTime=-1
  Constant : Constant  Value=fu0/BP0
  Constant1 : Constant  Value=V_DB
  Constant2 : Constant  Value=CL_PD_DS
  Constant3 : Constant  Value=beta
  Constant5 : Constant  Value=Q_kidney0
  Constant6 : Constant  Value=gamma
  Constant7 : Constant  Value=fu_k
  Divide1 : Product  Inputs=/*
  Integrator : Integrator
  Product{,1..3,5} (5 alike) : Product  RndMeth=Zero
  Product6 : Product  Inputs=4  RndMeth=Zero
  Saturation : Saturate  UpperLimit=1000000000  LowerLimit=0
  Subtract : Sum
  Subtract1 : Sum
  Sum : Sum  Inputs=+-|
  scope : Scope
  Out1 : Outport
  wires:
  Integrator/1 -> Product2/2, Product6/4, Saturation/1, scope/1, C_DB/1
  Sum/1 -> Divide1/2
  Saturation/1 -> Out1/1
  Constant7/1 -> Product1/1
  Product1/1 -> Product3/1
  Constant5/1 -> Product2/1, Product/1
  Product3/1 -> Subtract/1
  Product/1 -> Subtract/2
  Constant1/1 -> Divide1/1
  Subtract/1 -> Sum/1
  Divide1/1 -> Integrator/1
  Constant3/1 -> Product5/1
  Constant2/1 -> Product6/3, Product5/2
  Product5/1 -> Product3/2
  Subtract1/1 -> Sum/2
  C_Cell/1 -> Product1/2
  C_Blood/1 -> Product/2
  Constant/1 -> Product6/1
  Product2/1 -> Subtract1/1
  Constant6/1 -> Product6/2
  Product6/1 -> Subtract1/2

== system Huang_Isoherranen_Mechanistic_Kidney_Model/Huang Isoherranen Mechanistic Kidney Model/Kidney/Distal cell ==
  C_tube : Inport
  C_blood : Inport  Port=2
  C_DC : ToWorkspace  VariableName=C_DC  SampleTime=-1
  Constant : Constant  Value=CL_PD_DS
  Constant1 : Constant  Value=V_DC
  Constant2 : Constant  Value=CL_PD_DS
  Constant3 : Constant  Value=fu0/BP0
  Constant4 : Constant  Value=gamma
  Constant6 : Constant  Value=alpha_6
  Constant7 : Constant  Value=fu_k
  Constant8 : Constant  Value=beta
  Divide2 : Product  Inputs=/*
  Integrator : Integrator
  Product1 : Product  Inputs=3  RndMeth=Zero
  Product2 : Product  RndMeth=Zero
  Product3 : Product  Inputs=3  RndMeth=Zero
  Product4 : Product  RndMeth=Zero
  Product7 : Product  Inputs=3  RndMeth=Zero
  Subtract : Sum
  Subtract1 : Sum
  Sum : Sum  Inputs=+-|
  scope : Scope
  Out1 : Outport
  wires:
  Integrator/1 -> Product2/2, Out1/1, scope/1, C_DC/1
  C_tube/1 -> Product1/2
  Constant/1 -> Subtract1/2, Product1/1
  Constant2/1 -> Subtract1/1, Product3/1
  Constant4/1 -> Product3/2
  Subtract/1 -> Sum/1
  Product3/1 -> Subtract/2
  C_blood/1 -> Product4/1
  Constant3/1 -> Product4/2
  Product4/1 -> Product3/3
  Constant6/1 -> Product1/3
  Product1/1 -> Subtract/1
  Sum/1 -> Divide2/2
  Constant1/1 -> Divide2/1
  Divide2/1 -> Integrator/1
  Product2/1 -> Product7/3
  Constant7/1 -> Product2/1
  Constant8/1 -> Product7/2
  Subtract1/1 -> Product7/1
  Product7/1 -> Sum/2

== system Huang_Isoherranen_Mechanistic_Kidney_Model/Huang Isoherranen Mechanistic Kidney Model/Kidney/Distal tube ==
  C_Tube : Inport
  C_Cell : Inport  Port=2
  C_DT : ToWorkspace  VariableName=C_DT  SampleTime=-1
  Constant1 : Constant  Value=V_DT
  Constant2 : Constant  Value=CL_PD_DS
  Constant3 : Constant  Value=beta
  Constant4 : Constant  Value=Q_GFR/120*Q_connectingtubule
  Constant5 : Constant  Value=Q_GFR/120*24
  Constant6 : Constant  Value=alpha_6
  Constant7 : Constant  Value=fu_k
  Divide1 : Product  Inputs=/*
  Integrator : Integrator
  Product{,1..3,5} (5 alike) : Product  RndMeth=Zero
  Product6 : Product  Inputs=3  RndMeth=Zero
  Saturation : Saturate  UpperLimit=1000000000  LowerLimit=0
  Subtract : Sum
  Subtract1 : Sum
  Sum : Sum  Inputs=+-|
  scope : Scope
  Out1 : Outport
  wires:
  Integrator/1 -> Product2/2, Product6/3, Saturation/1, scope/1, C_DT/1
  Sum/1 -> Divide1/2
  Saturation/1 -> Out1/1
  C_Tube/1 -> Product/2
  Constant7/1 -> Product1/1
  C_Cell/1 -> Product1/2
  Product1/1 -> Product3/1
  Constant5/1 -> Product/1
  Product3/1 -> Subtract/1
  Product/1 -> Subtract/2
  Constant1/1 -> Divide1/1
  Subtract/1 -> Sum/1
  Divide1/1 -> Integrator/1
  Constant4/1 -> Product2/1
  Constant3/1 -> Product5/1
  Constant2/1 -> Product6/2, Product5/2
  Product5/1 -> Product3/2
  Constant6/1 -> Product6/1
  Product6/1 -> Subtract1/1
  Product2/1 -> Subtract1/2
  Subtract1/1 -> Sum/2

== system Huang_Isoherranen_Mechanistic_Kidney_Model/Huang Isoherranen Mechanistic Kidney Model/Kidney/Henle blood ==
  C_Cell : Inport
  C_Blood : Inport  Port=2
  C_HB : ToWorkspace  VariableName=C_HB_2  SampleTime=-1
  Constant : Constant  Value=fu0/BP0
  Constant1 : Constant  Value=V_HB
  Constant2 : Constant  Value=CL_PD_LH
  Constant3 : Constant  Value=beta
  Constant5 : Constant  Value=Q_kidney0
  Constant6 : Constant  Value=gamma
  Constant7 : Constant  Value=fu_k
  Divide1 : Product  Inputs=/*
  Integrator : Integrator
  Product{,1..3,5} (5 alike) : Product  RndMeth=Zero
  Product6 : Product  Inputs=4  RndMeth=Zero
  Saturation : Saturate  UpperLimit=1000000000  LowerLimit=0
  Subtract : Sum
  Subtract1 : Sum
  Sum : Sum  Inputs=+-|
  scope : Scope
  Out1 : Outport
  wires:
  Integrator/1 -> Product2/2, Product6/4, Saturation/1, scope/1, C_HB/1
  Sum/1 -> Divide1/2
  Saturation/1 -> Out1/1
  Constant7/1 -> Product1/1
  Product1/1 -> Product3/1
  Constant5/1 -> Product2/1, Product/1
  Product3/1 -> Subtract/1
  Product/1 -> Subtract/2
  Constant1/1 -> Divide1/1
  Subtract/1 -> Sum/1
  Divide1/1 -> Integrator/1
  Constant3/1 -> Product5/1
  Constant2/1 -> Product6/3, Product5/2
  Product5/1 -> Product3/2
  Subtract1/1 -> Sum/2
  C_Cell/1 -> Product1/2
  C_Blood/1 -> Product/2
  Constant/1 -> Product6/1
  Product2/1 -> Subtract1/1
  Constant6/1 -> Product6/2
  Product6/1 -> Subtract1/2

== system Huang_Isoherranen_Mechanistic_Kidney_Model/Huang Isoherranen Mechanistic Kidney Model/Kidney/Henle blood1 ==
  C_Cell : Inport
  C_Blood : Inport  Port=2
  C_HB : ToWorkspace  VariableName=C_HB  SampleTime=-1
  Constant : Constant  Value=fu0/BP0
  Constant1 : Constant  Value=V_HB
  Constant2 : Constant  Value=CL_PD_LH
  Constant3 : Constant  Value=beta
  Constant5 : Constant  Value=Q_kidney0
  Constant6 : Constant  Value=gamma
  Constant7 : Constant  Value=fu_k
  Divide1 : Product  Inputs=/*
  Integrator : Integrator
  Product{,1..3,5} (5 alike) : Product  RndMeth=Zero
  Product6 : Product  Inputs=4  RndMeth=Zero
  Saturation : Saturate  UpperLimit=1000000000  LowerLimit=0
  Subtract : Sum
  Subtract1 : Sum
  Sum : Sum  Inputs=+-|
  scope : Scope
  Out1 : Outport
  wires:
  Integrator/1 -> Product2/2, Product6/4, Saturation/1, scope/1, C_HB/1
  Sum/1 -> Divide1/2
  Saturation/1 -> Out1/1
  Constant7/1 -> Product1/1
  Product1/1 -> Product3/1
  Constant5/1 -> Product2/1, Product/1
  Product3/1 -> Subtract/1
  Product/1 -> Subtract/2
  Constant1/1 -> Divide1/1
  Subtract/1 -> Sum/1
  Divide1/1 -> Integrator/1
  Constant3/1 -> Product5/1
  Constant2/1 -> Product6/3, Product5/2
  Product5/1 -> Product3/2
  Subtract1/1 -> Sum/2
  C_Cell/1 -> Product1/2
  C_Blood/1 -> Product/2
  Constant/1 -> Product6/1
  Product2/1 -> Subtract1/1
  Constant6/1 -> Product6/2
  Product6/1 -> Subtract1/2

== system Huang_Isoherranen_Mechanistic_Kidney_Model/Huang Isoherranen Mechanistic Kidney Model/Kidney/Henle cell ==
  C_tube : Inport
  C_blood : Inport  Port=2
  C_HC : ToWorkspace  VariableName=C_HC_2  SampleTime=-1
  Constant : Constant  Value=CL_PD_LH
  Constant1 : Constant  Value=V_HC
  Constant2 : Constant  Value=CL_PD_LH
  Constant3 : Constant  Value=fu0/BP0
  Constant4 : Constant  Value=gamma
  Constant6 : Constant  Value=alpha_5
  Constant7 : Constant  Value=fu_k
  Constant8 : Constant  Value=beta
  Divide2 : Product  Inputs=/*
  Integrator : Integrator
  Product1 : Product  Inputs=3  RndMeth=Zero
  Product2 : Product  RndMeth=Zero
  Product3 : Product  Inputs=3  RndMeth=Zero
  Product4 : Product  RndMeth=Zero
  Product7 : Product  Inputs=3  RndMeth=Zero
  Subtract : Sum
  Subtract1 : Sum
  Sum : Sum  Inputs=+-|
  scope : Scope
  Out1 : Outport
  wires:
  Integrator/1 -> Product2/2, Out1/1, scope/1, C_HC/1
  C_tube/1 -> Product1/2
  Constant/1 -> Subtract1/2, Product1/1
  Constant2/1 -> Subtract1/1, Product3/1
  Constant4/1 -> Product3/2
  Subtract/1 -> Sum/1
  Product3/1 -> Subtract/2
  C_blood/1 -> Product4/1
  Constant3/1 -> Product4/2
  Product4/1 -> Product3/3
  Constant6/1 -> Product1/3
  Product1/1 -> Subtract/1
  Sum/1 -> Divide2/2
  Constant1/1 -> Divide2/1
  Divide2/1 -> Integrator/1
  Product2/1 -> Product7/3
  Constant7/1 -> Product2/1
  Constant8/1 -> Product7/2
  Subtract1/1 -> Product7/1
  Product7/1 -> Sum/2

== system Huang_Isoherranen_Mechanistic_Kidney_Model/Huang Isoherranen Mechanistic Kidney Model/Kidney/Henle cell1 ==
  C_tube : Inport
  C_blood : Inport  Port=2
  C_HC : ToWorkspace  VariableName=C_HC  SampleTime=-1
  Constant : Constant  Value=CL_PD_LH
  Constant1 : Constant  Value=V_HC
  Constant2 : Constant  Value=CL_PD_LH
  Constant3 : Constant  Value=fu0/BP0
  Constant4 : Constant  Value=gamma
  Constant6 : Constant  Value=alpha_4
  Constant7 : Constant  Value=fu_k
  Constant8 : Constant  Value=beta
  Divide2 : Product  Inputs=/*
  Integrator : Integrator
  Product1 : Product  Inputs=3  RndMeth=Zero
  Product2 : Product  RndMeth=Zero
  Product3 : Product  Inputs=3  RndMeth=Zero
  Product4 : Product  RndMeth=Zero
  Product7 : Product  Inputs=3  RndMeth=Zero
  Subtract : Sum
  Subtract1 : Sum
  Sum : Sum  Inputs=+-|
  scope : Scope
  Out1 : Outport
  wires:
  Integrator/1 -> Product2/2, Out1/1, scope/1, C_HC/1
  C_tube/1 -> Product1/2
  Constant/1 -> Subtract1/2, Product1/1
  Constant2/1 -> Subtract1/1, Product3/1
  Constant4/1 -> Product3/2
  Subtract/1 -> Sum/1
  Product3/1 -> Subtract/2
  C_blood/1 -> Product4/1
  Constant3/1 -> Product4/2
  Product4/1 -> Product3/3
  Constant6/1 -> Product1/3
  Product1/1 -> Subtract/1
  Sum/1 -> Divide2/2
  Constant1/1 -> Divide2/1
  Divide2/1 -> Integrator/1
  Product2/1 -> Product7/3
  Constant7/1 -> Product2/1
  Constant8/1 -> Product7/2
  Subtract1/1 -> Product7/1
  Product7/1 -> Sum/2

== system Huang_Isoherranen_Mechanistic_Kidney_Model/Huang Isoherranen Mechanistic Kidney Model/Kidney/Initial collecting tubule ==
  C_Tube : Inport
  C_Cell : Inport  Port=2
  C_CDT_2 : ToWorkspace  VariableName=C_CDT_2  SampleTime=-1
  Constant1 : Constant  Value=V_CDT
  Constant2 : Constant  Value=CL_PD_CD
  Constant3 : Constant  Value=beta
  Constant4 : Constant  Value=Q_GFR/120*Q_corticalCD
  Constant5 : Constant  Value=Q_GFR/120*Q_initialCD
  Constant6 : Constant  Value=alpha_8
  Constant7 : Constant  Value=fu_k
  Divide1 : Product  Inputs=/*
  Integrator : Integrator
  Product{,1..3,5} (5 alike) : Product  RndMeth=Zero
  Product6 : Product  Inputs=3  RndMeth=Zero
  Saturation : Saturate  UpperLimit=1000000000  LowerLimit=0
  Subtract : Sum
  Subtract1 : Sum
  Sum : Sum  Inputs=+-|
  scope : Scope
  Out1 : Outport
  wires:
  Integrator/1 -> Product2/2, Product6/3, Saturation/1, scope/1, C_CDT_2/1
  Sum/1 -> Divide1/2
  Saturation/1 -> Out1/1
  C_Tube/1 -> Product/2
  Constant7/1 -> Product1/1
  C_Cell/1 -> Product1/2
  Product1/1 -> Product3/1
  Constant5/1 -> Product/1
  Product3/1 -> Subtract/1
  Product/1 -> Subtract/2
  Constant1/1 -> Divide1/1
  Subtract/1 -> Sum/1
  Divide1/1 -> Integrator/1
  Constant4/1 -> Product2/1
  Constant3/1 -> Product5/1
  Constant2/1 -> Product6/2, Product5/2
  Product5/1 -> Product3/2
  Constant6/1 -> Product6/1
  Product6/1 -> Subtract1/1
  Product2/1 -> Subtract1/2
  Subtract1/1 -> Sum/2

== system Huang_Isoherranen_Mechanistic_Kidney_Model/Huang Isoherranen Mechanistic Kidney Model/Kidney/Medullary CD ==
  C_Tube : Inport
  C_Cell : Inport  Port=2
  C_CDT_4 : ToWorkspace  VariableName=C_CDT_4  SampleTime=-1
  Constant1 : Constant  Value=V_CDT
  Constant2 : Constant  Value=CL_PD_CD
  Constant3 : Constant  Value=beta
  Constant4 : Constant  Value=Q_GFR/120*Q_papillary
  Constant5 : Constant  Value=Q_GFR/120*Q_medullaryCD
  Constant6 : Constant  Value=alpha_10
  Constant7 : Constant  Value=fu_k
  Divide1 : Product  Inputs=/*
  Integrator : Integrator
  Product{,1..3,5} (5 alike) : Product  RndMeth=Zero
  Product6 : Product  Inputs=3  RndMeth=Zero
  Saturation : Saturate  UpperLimit=1000000000  LowerLimit=0
  Subtract : Sum
  Subtract1 : Sum
  Sum : Sum  Inputs=+-|
  scope : Scope
  Out1 : Outport
  wires:
  Integrator/1 -> Product2/2, Product6/3, Saturation/1, scope/1, C_CDT_4/1
  Sum/1 -> Divide1/2
  Saturation/1 -> Out1/1
  C_Tube/1 -> Product/2
  Constant7/1 -> Product1/1
  C_Cell/1 -> Product1/2
  Product1/1 -> Product3/1
  Constant5/1 -> Product/1
  Product3/1 -> Subtract/1
  Product/1 -> Subtract/2
  Constant1/1 -> Divide1/1
  Subtract/1 -> Sum/1
  Divide1/1 -> Integrator/1
  Constant4/1 -> Product2/1
  Constant3/1 -> Product5/1
  Constant2/1 -> Product6/2, Product5/2
  Product5/1 -> Product3/2
  Constant6/1 -> Product6/1
  Product6/1 -> Subtract1/1
  Product2/1 -> Subtract1/2
  Subtract1/1 -> Sum/2

== system Huang_Isoherranen_Mechanistic_Kidney_Model/Huang Isoherranen Mechanistic Kidney Model/Kidney/Papillary duct ==
  C_Tube : Inport
  C_Cell : Inport  Port=2
  C_CDT_4 : ToWorkspace  VariableName=C_CDT_5  SampleTime=-1
  Constant1 : Constant  Value=V_CDT
  Constant2 : Constant  Value=CL_PD_CD
  Constant3 : Constant  Value=beta
  Constant4 : Constant  Value=Q_GFR/120*Q_urine
  Constant5 : Constant  Value=Q_GFR/120*Q_papillary
  Constant6 : Constant  Value=alpha_11
  Constant7 : Constant  Value=fu_k
  Divide1 : Product  Inputs=/*
  Integrator : Integrator
  Product{,1..3,5} (5 alike) : Product  RndMeth=Zero
  Product6 : Product  Inputs=3  RndMeth=Zero
  Saturation : Saturate  UpperLimit=1000000000  LowerLimit=0
  Subtract : Sum
  Subtract1 : Sum
  Sum : Sum  Inputs=+-|
  scope : Scope
  Out1 : Outport
  wires:
  Integrator/1 -> Product2/2, Product6/3, Saturation/1, scope/1, C_CDT_4/1
  Sum/1 -> Divide1/2
  Saturation/1 -> Out1/1
  C_Tube/1 -> Product/2
  Constant7/1 -> Product1/1
  C_Cell/1 -> Product1/2
  Product1/1 -> Product3/1
  Constant5/1 -> Product/1
  Product3/1 -> Subtract/1
  Product/1 -> Subtract/2
  Constant1/1 -> Divide1/1
  Subtract/1 -> Sum/1
  Divide1/1 -> Integrator/1
  Constant4/1 -> Product2/1
  Constant3/1 -> Product5/1
  Constant2/1 -> Product6/2, Product5/2
  Product5/1 -> Product3/2
  Constant6/1 -> Product6/1
  Product6/1 -> Subtract1/1
  Product2/1 -> Subtract1/2
  Subtract1/1 -> Sum/2
